simulink model "model"  (R2022a)
settings: Solver=VariableStepAuto  StartTime=0.0  StopTime=100  RelTol=1e-3
undefined symbols (not defined in the file): A0, A1, B0, B1, C0, C1, G, K, Ki, Kx, L, l, L0
settings Model: Creator=jhocq  LastModifiedBy=JHOCQ
settings SolverCC: AlgebraicLoopSolver=TrustRegion
settings DebuggingCC: UnconnectedInputMsg=warning  UnconnectedOutputMsg=warning  UnconnectedLineMsg=warning  SFMachineParentedDataDiag=warning
settings RTWCC: DLArmComputeVersion=19.05

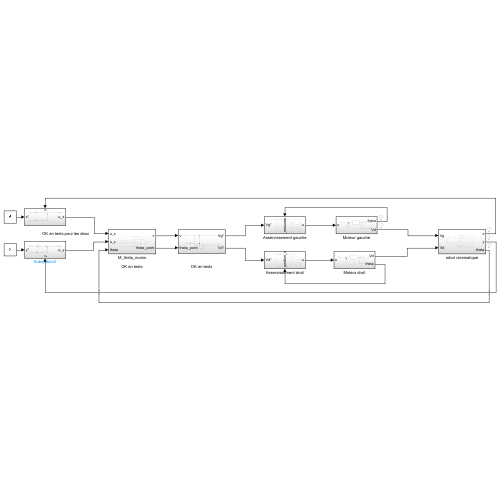
[thumbnail: Simulink's stored preview of the top-level diagram]
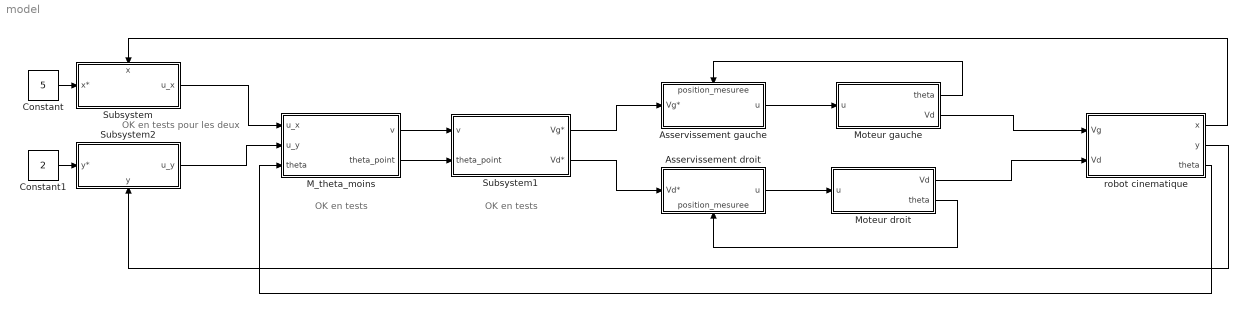
== system model ==
  note: OK en tests pour les deux
  note: OK en tests
  note: OK en tests
  Asservissement droit : Subsystem
      settings: PortSchema="{\"entries\":[{\"content\":{\"sides\":[{\"content\":{\"connectorIds\":[\"In1\"]},\"type\":\"ConnectorPlacement.EquallySpacedRectSide\",\"uuid\":\"34affdbf-5d75-4bee-a322-280e31ed4067\"},{\"content\":{\"connectorIds\":[\"Out1\"],\"side\":\"RIGHT\"},\"type\":\"ConnectorPlacement.EquallySpacedRectSide\",\"uuid\":\"c24ccca8-e7ae-4acc-ac9f-82cb89bd5926\"},{\"content\":{\"connectorIds\":[],\"side\":\"TOP\"},\"type\":\"ConnectorPlacement.EquallySpacedRectSide\",\"uuid\":\"edb210ed-4fa8-422f-a5d5-5fbb66d57dd6\"},{\"content\":{\"connectorIds\":[\"In2\"],\"side\":\"BOTTOM\"},\"type\":\"ConnectorPlacement.EquallySpacedRectSide\",\"uuid\":\"957cfe47-833c-4a06-874b-fd027ee464dc\"},{\"content\":{\"connectorIds\":[],\"side\":\"HIDDEN\"},\"type\":\"ConnectorPlacement.EquallySpacedRectSide\",\"uuid\":\"109f9272-0331-4963-a029-781066042169\"}]},\"type\":\"ConnectorPlacement.EquallySpacedConnector\",\"uuid\":\"ee06e29f-9d62-4172-95e8-826ec0e998b9\"}],\"packageUris\":[\"http://schema.mathworks.com/mf0/Connector/R2020b\"],\"version\":\"1.0\"}"
  Asservissement gauche : Subsystem
      settings: PortSchema="{\"entries\":[{\"content\":{\"sides\":[{\"content\":{\"connectorIds\":[\"In1\"]},\"type\":\"ConnectorPlacement.EquallySpacedRectSide\",\"uuid\":\"34affdbf-5d75-4bee-a322-280e31ed4067\"},{\"content\":{\"connectorIds\":[\"Out1\"],\"side\":\"RIGHT\"},\"type\":\"ConnectorPlacement.EquallySpacedRectSide\",\"uuid\":\"c24ccca8-e7ae-4acc-ac9f-82cb89bd5926\"},{\"content\":{\"connectorIds\":[\"In2\"],\"side\":\"TOP\"},\"type\":\"ConnectorPlacement.EquallySpacedRectSide\",\"uuid\":\"edb210ed-4fa8-422f-a5d5-5fbb66d57dd6\"},{\"content\":{\"connectorIds\":[],\"side\":\"BOTTOM\"},\"type\":\"ConnectorPlacement.EquallySpacedRectSide\",\"uuid\":\"957cfe47-833c-4a06-874b-fd027ee464dc\"},{\"content\":{\"connectorIds\":[],\"side\":\"HIDDEN\"},\"type\":\"ConnectorPlacement.EquallySpacedRectSide\",\"uuid\":\"109f9272-0331-4963-a029-781066042169\"}]},\"type\":\"ConnectorPlacement.EquallySpacedConnector\",\"uuid\":\"ee06e29f-9d62-4172-95e8-826ec0e998b9\"}],\"packageUris\":[\"http://schema.mathworks.com/mf0/Connector/R2020b\"],\"version\":\"1.0\"}"
  Constant : Constant  Value=5
  Constant1 : Constant  Value=2
  M_theta_moins : Subsystem
  Moteur droit : Subsystem
  Moteur gauche : Subsystem
  Subsystem : Subsystem
      settings: PortSchema="{\"entries\":[{\"content\":{\"sides\":[{\"content\":{\"connectorIds\":[\"In1\"]},\"type\":\"ConnectorPlacement.EquallySpacedRectSide\",\"uuid\":\"338121f5-c05f-4735-9fae-09ea2fac0aa8\"},{\"content\":{\"connectorIds\":[\"Out1\"],\"side\":\"RIGHT\"},\"type\":\"ConnectorPlacement.EquallySpacedRectSide\",\"uuid\":\"4e5e0544-0927-46bc-93f3-46a3a0a84001\"},{\"content\":{\"connectorIds\":[\"In2\"],\"side\":\"TOP\"},\"type\":\"ConnectorPlacement.EquallySpacedRectSide\",\"uuid\":\"e6da10fa-0f76-4df7-a8fb-a988bc5ccb33\"},{\"content\":{\"connectorIds\":[],\"side\":\"HIDDEN\"},\"type\":\"ConnectorPlacement.EquallySpacedRectSide\",\"uuid\":\"904212ea-ca19-48d6-920f-a5e1b3dde1fc\"}]},\"type\":\"ConnectorPlacement.EquallySpacedConnector\",\"uuid\":\"e42c5e64-dc68-42eb-86fa-c75e656ddd55\"}],\"packageUris\":[\"http://schema.mathworks.com/mf0/Connector/R2020b\"],\"version\":\"1.0\"}"
  Subsystem1 : Subsystem
  Subsystem2 : Subsystem
      settings: PortSchema="{\"entries\":[{\"content\":{\"sides\":[{\"content\":{\"connectorIds\":[\"In1\"]},\"type\":\"ConnectorPlacement.EquallySpacedRectSide\",\"uuid\":\"338121f5-c05f-4735-9fae-09ea2fac0aa8\"},{\"content\":{\"connectorIds\":[\"Out1\"],\"side\":\"RIGHT\"},\"type\":\"ConnectorPlacement.EquallySpacedRectSide\",\"uuid\":\"4e5e0544-0927-46bc-93f3-46a3a0a84001\"},{\"content\":{\"connectorIds\":[],\"side\":\"TOP\"},\"type\":\"ConnectorPlacement.EquallySpacedRectSide\",\"uuid\":\"e6da10fa-0f76-4df7-a8fb-a988bc5ccb33\"},{\"content\":{\"connectorIds\":[\"In2\"],\"side\":\"BOTTOM\"},\"type\":\"ConnectorPlacement.EquallySpacedRectSide\",\"uuid\":\"13297936-a58e-4a97-9ae4-702edafcee13\"},{\"content\":{\"connectorIds\":[],\"side\":\"HIDDEN\"},\"type\":\"ConnectorPlacement.EquallySpacedRectSide\",\"uuid\":\"904212ea-ca19-48d6-920f-a5e1b3dde1fc\"}]},\"type\":\"ConnectorPlacement.EquallySpacedConnector\",\"uuid\":\"e42c5e64-dc68-42eb-86fa-c75e656ddd55\"}],\"packageUris\":[\"http://schema.mathworks.com/mf0/Connector/R2020b\"],\"version\":\"1.0\"}"
  robot cinematique : Subsystem
  wires:
  Constant1/1 -> Subsystem2/1(y*)
  Constant/1 -> Subsystem/1(x*)
  robot cinematique/2(y) -> Subsystem2/2(y)
  Subsystem1/2(Vd*) -> Asservissement droit/1(Vd*)
  Asservissement droit/1(u) -> Moteur droit/1(u)
  Moteur droit/2(theta) -> Asservissement droit/2(position_mesuree)
  robot cinematique/1(x) -> Subsystem/2(x)
  Subsystem2/1(u_y) -> M_theta_moins/2(u_y)
  Subsystem/1(u_x) -> M_theta_moins/1(u_x)
  robot cinematique/3(theta) -> M_theta_moins/3(theta)
  M_theta_moins/1(v) -> Subsystem1/1(v)
  M_theta_moins/2(theta_point) -> Subsystem1/2(theta_point)
  Moteur gauche/2(Vd) -> robot cinematique/1(Vg)
  Moteur droit/1(Vd) -> robot cinematique/2(Vd)
  Asservissement gauche/1(u) -> Moteur gauche/1(u)
  Moteur gauche/1(theta) -> Asservissement gauche/2(position_mesuree)
  Subsystem1/1(Vg*) -> Asservissement gauche/1(Vg*)

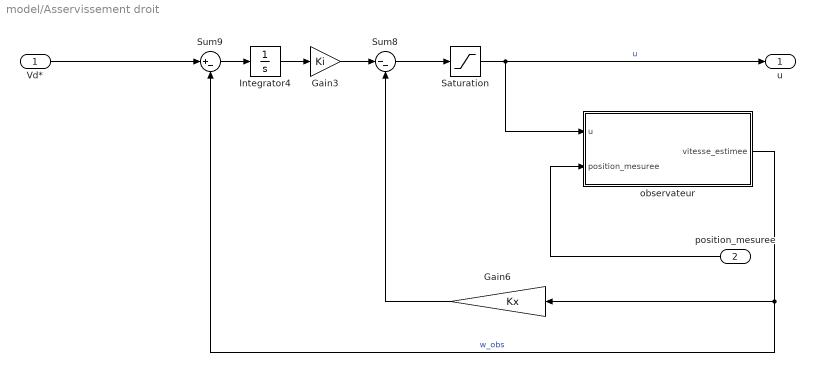
== system model/Asservissement droit ==
  Vd* : Inport
  position_mesuree : Inport  Port=2
  Gain3 : Gain  Gain=Ki
  Gain6 : Gain  Gain=Kx
  Integrator4 : Integrator
  Saturation : Saturate  UpperLimit=9  LowerLimit=-9
      settings: AttributesFormatString=[%<LowerLimit> %<UpperLimit>]
  Sum8 : Sum  Inputs=|--
  Sum9 : Sum  Inputs=|+-
  observateur : Subsystem
  u : Outport
  wires:
  Integrator4/1 -> Gain3/1
  Gain3/1 -> Sum8/1
  Vd*/1 -> Sum9/1
  Sum9/1 -> Integrator4/1
  Sum8/1 -> Saturation/1
  Saturation/1 -> observateur/1(u), u/1  "u"
  observateur/1(vitesse_estimee) -> Sum9/2, Gain6/1  "w_obs"
  Gain6/1 -> Sum8/2
  position_mesuree/1 -> observateur/2(position_mesuree)

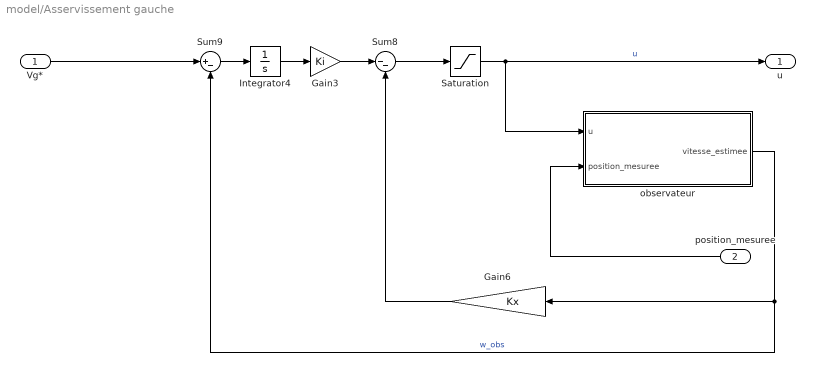
== system model/Asservissement gauche ==
  Vg* : Inport
  position_mesuree : Inport  Port=2
  Gain3 : Gain  Gain=Ki
  Gain6 : Gain  Gain=Kx
  Integrator4 : Integrator
  Saturation : Saturate  UpperLimit=9  LowerLimit=-9
      settings: AttributesFormatString=[%<LowerLimit> %<UpperLimit>]
  Sum8 : Sum  Inputs=|--
  Sum9 : Sum  Inputs=|+-
  observateur : Subsystem
  u : Outport
  wires:
  Integrator4/1 -> Gain3/1
  Gain3/1 -> Sum8/1
  Vg*/1 -> Sum9/1
  Sum9/1 -> Integrator4/1
  Sum8/1 -> Saturation/1
  Saturation/1 -> observateur/1(u), u/1  "u"
  observateur/1(vitesse_estimee) -> Sum9/2, Gain6/1  "w_obs"
  Gain6/1 -> Sum8/2
  position_mesuree/1 -> observateur/2(position_mesuree)

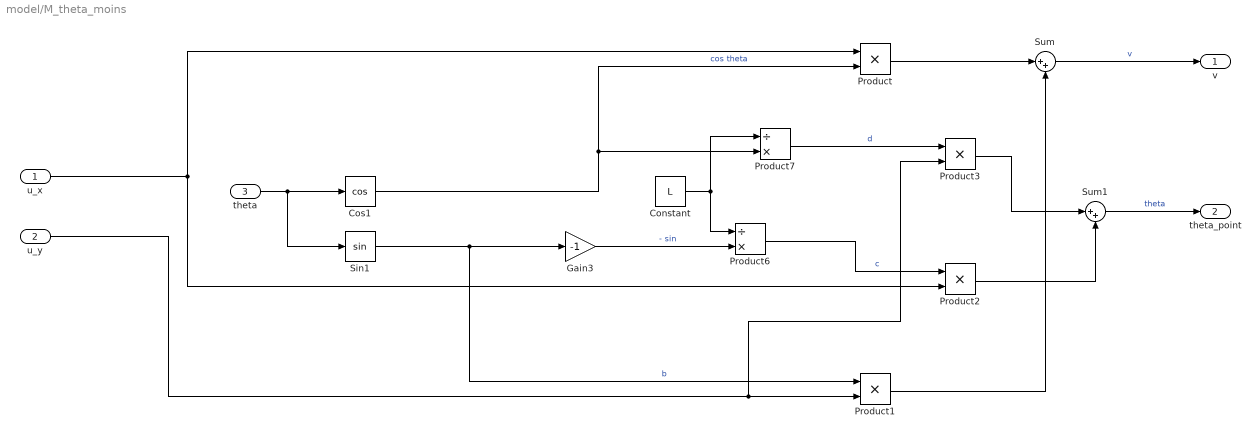
== system model/M_theta_moins ==
  u_x : Inport
  u_y : Inport  Port=2
  theta : Inport  Port=3
  Constant : Constant  Value=L
  Cos1 : Trigonometry  Operator=cos
  Gain3 : Gain  Gain=-1
  Product{,1..3} (4 alike) : Product
  Product6 : Product  Inputs=/*
  Product7 : Product  Inputs=/*
  Sin1 : Trigonometry
  Sum : Sum  Inputs=|++
  Sum1 : Sum  Inputs=|++
  v : Outport
  theta_point : Outport  Port=2
  wires:
  theta/1 -> Sin1/1, Cos1/1
  Sin1/1 -> Product1/1, Gain3/1  "b"
  Gain3/1 -> Product6/2  "- sin"
  Cos1/1 -> Product/2, Product7/2  "cos theta"
  Constant/1 -> Product6/1, Product7/1
  Product6/1 -> Product2/1  "c"
  Product7/1 -> Product3/1  "d"
  u_x/1 -> Product2/2, Product/1
  u_y/1 -> Product3/2, Product1/2
  Product/1 -> Sum/1
  Product1/1 -> Sum/2
  Sum/1 -> v/1  "v"
  Sum1/1 -> theta_point/1  "theta"
  Product2/1 -> Sum1/2
  Product3/1 -> Sum1/1

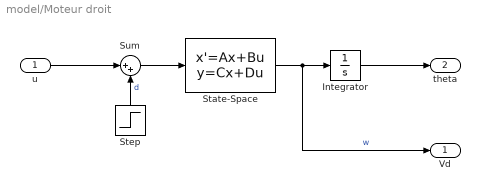
== system model/Moteur droit ==
  u : Inport
  Integrator : Integrator
  State-Space : StateSpace  A=A1  B=B1  C=C1  D=0  InitialCondition=0
  Step : Step  Time=5  SampleTime=0
  Sum : Sum  Inputs=|++
  Vd : Outport
  theta : Outport  Port=2
  wires:
  u/1 -> Sum/1
  Step/1 -> Sum/2  "d"
  Sum/1 -> State-Space/1
  State-Space/1 -> Vd/1, Integrator/1  "w"
  Integrator/1 -> theta/1

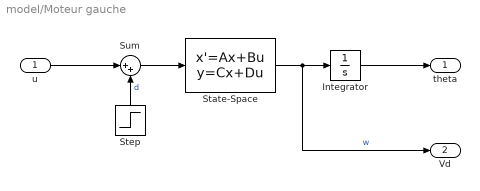
== system model/Moteur gauche ==
  u : Inport
  Integrator : Integrator
  State-Space : StateSpace  A=A1  B=B1  C=C1  D=0  InitialCondition=0
  Step : Step  Time=5  SampleTime=0
  Sum : Sum  Inputs=|++
  theta : Outport
  Vd : Outport  Port=2
  wires:
  u/1 -> Sum/1
  Step/1 -> Sum/2  "d"
  Sum/1 -> State-Space/1
  State-Space/1 -> Vd/1, Integrator/1  "w"
  Integrator/1 -> theta/1

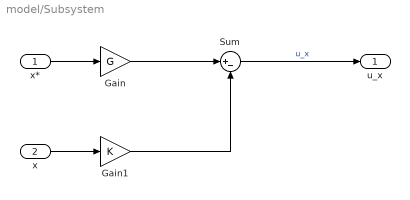
== system model/Subsystem ==
  x* : Inport
  x : Inport  Port=2
  Gain : Gain  Gain=G
  Gain1 : Gain  Gain=K
  Sum : Sum  Inputs=|+-
  u_x : Outport
  wires:
  Sum/1 -> u_x/1  "u_x"
  x*/1 -> Gain/1
  Gain/1 -> Sum/1
  x/1 -> Gain1/1
  Gain1/1 -> Sum/2

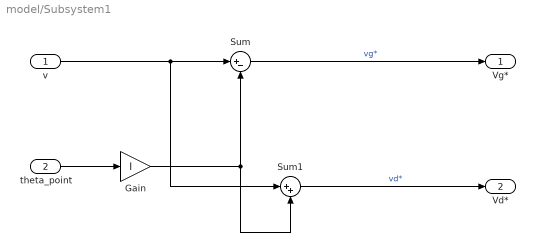
== system model/Subsystem1 ==
  v : Inport
  theta_point : Inport  Port=2
  Gain : Gain  Gain=l
  Sum : Sum  Inputs=|+-
  Sum1 : Sum  Inputs=|++
  Vg* : Outport
  Vd* : Outport  Port=2
  wires:
  v/1 -> Sum1/1, Sum/1
  theta_point/1 -> Gain/1
  Sum/1 -> Vg*/1  "vg*"
  Gain/1 -> Sum1/2, Sum/2
  Sum1/1 -> Vd*/1  "vd*"

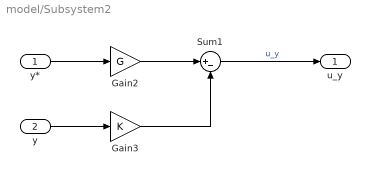
== system model/Subsystem2 ==
  y* : Inport
  y : Inport  Port=2
  Gain2 : Gain  Gain=G
  Gain3 : Gain  Gain=K
  Sum1 : Sum  Inputs=|+-
  u_y : Outport
  wires:
  y*/1 -> Gain2/1
  y/1 -> Gain3/1
  Gain2/1 -> Sum1/1
  Gain3/1 -> Sum1/2
  Sum1/1 -> u_y/1  "u_y"

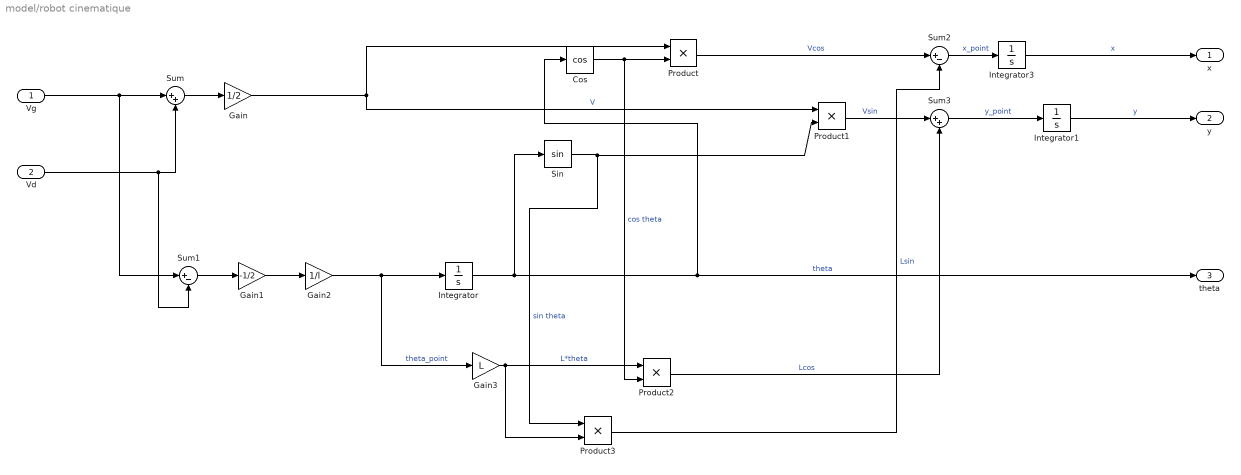
== system model/robot cinematique ==
  Vg : Inport
  Vd : Inport  Port=2
  Cos : Trigonometry  Operator=cos
  Gain : Gain  Gain=1/2
  Gain1 : Gain  Gain=-1/2
  Gain2 : Gain  Gain=1/l
  Gain3 : Gain  Gain=L
  Integrator : Integrator
  Integrator1 : Integrator
  Integrator3 : Integrator
  Product{,1..3} (4 alike) : Product
  Sin : Trigonometry
  Sum : Sum  Inputs=|++
  Sum1 : Sum  Inputs=|+-
  Sum2 : Sum  Inputs=|+-
  Sum3 : Sum  Inputs=|++
  x : Outport
  y : Outport  Port=2
  theta : Outport  Port=3
  wires:
  Vg/1 -> Sum1/1, Sum/1
  Vd/1 -> Sum/2, Sum1/2
  Sum/1 -> Gain/1
  Gain/1 -> Product1/1, Product/1  "V"
  Sum1/1 -> Gain1/1
  Gain1/1 -> Gain2/1
  Gain2/1 -> Gain3/1, Integrator/1  "theta_point"
  Integrator/1 -> Cos/1, theta/1, Sin/1  "theta"
  Integrator3/1 -> x/1  "x"
  Gain3/1 -> Product3/2, Product2/1  "L*theta"
  Integrator1/1 -> y/1  "y"
  Cos/1 -> Product2/2, Product/2  "cos theta"
  Sin/1 -> Product3/1, Product1/2  "sin theta"
  Product/1 -> Sum2/1  "Vcos"
  Product1/1 -> Sum3/1  "Vsin"
  Product2/1 -> Sum3/2  "Lcos"
  Sum2/1 -> Integrator3/1  "x_point"
  Sum3/1 -> Integrator1/1  "y_point"
  Product3/1 -> Sum2/2  "Lsin"

== system model/Asservissement droit/observateur ==
  u : Inport
  position_mesuree : Inport  Port=2
  Selector : Selector  InputPortWidth=3  IndexOptions=Index vector (dialog)  Indices=1  OutputSizes=1
  Subsystem : Subsystem
  vitesse_estimee : Outport
  wires:
  u/1 -> Subsystem/2(u)  "x"
  position_mesuree/1 -> Subsystem/1(y)
  Selector/1 -> vitesse_estimee/1  "w*"
  Subsystem/1(x_est1) -> Selector/1  "x_est"

== system model/Asservissement gauche/observateur ==
  u : Inport
  position_mesuree : Inport  Port=2
  Selector : Selector  InputPortWidth=3  IndexOptions=Index vector (dialog)  Indices=1  OutputSizes=1
  Subsystem : Subsystem
  vitesse_estimee : Outport
  wires:
  u/1 -> Subsystem/2(u)  "x"
  position_mesuree/1 -> Subsystem/1(y)
  Selector/1 -> vitesse_estimee/1  "w*"
  Subsystem/1(x_est1) -> Selector/1  "x_est"

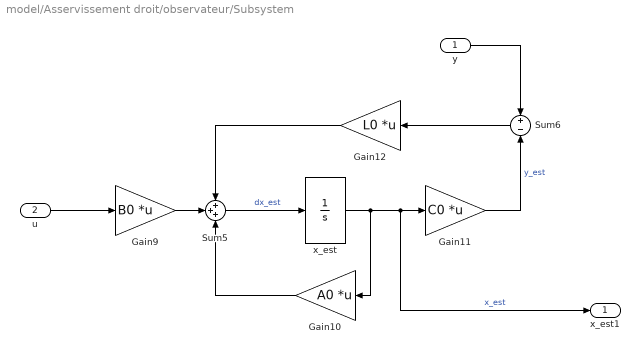
== system model/Asservissement droit/observateur/Subsystem ==
  y : Inport
  u : Inport  Port=2
  Gain10 : Gain  Gain=A0  Multiplication=Matrix(K*u)
  Gain11 : Gain  Gain=C0  Multiplication=Matrix(K*u)
  Gain12 : Gain  Gain=L0  Multiplication=Matrix(K*u)
  Gain9 : Gain  Gain=B0  Multiplication=Matrix(K*u)
  Sum5 : Sum  Inputs=+++
  Sum6 : Sum  Inputs=+-
  x_est : Integrator
  x_est1 : Outport
  wires:
  y/1 -> Sum6/1
  Sum5/1 -> x_est/1  "dx_est"
  Gain12/1 -> Sum5/1
  Sum6/1 -> Gain12/1
  Gain9/1 -> Sum5/2
  Gain11/1 -> Sum6/2  "y_est"
  Gain10/1 -> Sum5/3
  u/1 -> Gain9/1
  x_est/1 -> x_est1/1, Gain11/1, Gain10/1  "x_est"

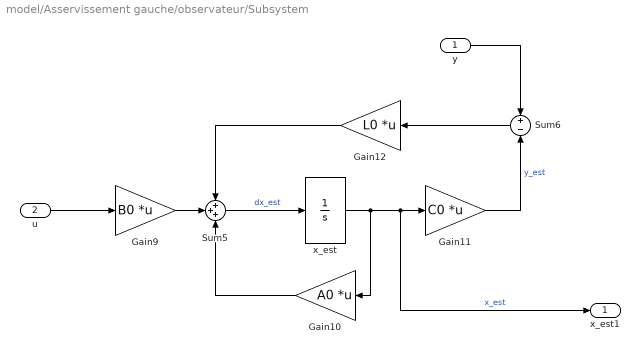
== system model/Asservissement gauche/observateur/Subsystem ==
  y : Inport
  u : Inport  Port=2
  Gain10 : Gain  Gain=A0  Multiplication=Matrix(K*u)
  Gain11 : Gain  Gain=C0  Multiplication=Matrix(K*u)
  Gain12 : Gain  Gain=L0  Multiplication=Matrix(K*u)
  Gain9 : Gain  Gain=B0  Multiplication=Matrix(K*u)
  Sum5 : Sum  Inputs=+++
  Sum6 : Sum  Inputs=+-
  x_est : Integrator
  x_est1 : Outport
  wires:
  y/1 -> Sum6/1
  Sum5/1 -> x_est/1  "dx_est"
  Gain12/1 -> Sum5/1
  Sum6/1 -> Gain12/1
  Gain9/1 -> Sum5/2
  Gain11/1 -> Sum6/2  "y_est"
  Gain10/1 -> Sum5/3
  u/1 -> Gain9/1
  x_est/1 -> x_est1/1, Gain11/1, Gain10/1  "x_est"
